simulink library "GOcontroll_Generic"  (R2023b)
settings: Solver=ode45  StartTime=0.0  StopTime=10.0  RelTol=1e-3  EnableMultiTasking=on
undefined symbols (not defined in the file or in its folder): C_CatOutPos, C_Cb1Pt10, Cb1Pt10_RAW_ERR_HIGH, Cb1Pt10_RAW_ERR_LOW, Cb1Pt10_SIG_ERR_HIGH, Cb1Pt10_SIG_ERR_LOW, Cb1Pt10_SIG_WAR_HIGH, Cb1Pt10_SIG_WAR_LOW, M_CatOutPos, Pres_0_20_bar_500_4500_mv_inv, SensorSignalSimulation, signal_x_RAW_ERR_HIGH, signal_x_RAW_ERR_LOW, signal_x_SIG_ERR_HIGH, signal_x_SIG_ERR_LOW, signal_x_SIG_WAR_HIGH, signal_x_SIG_WAR_LOW, signal_x_SPN, Valve1_ACTIVE_DUTY_CYCLE, Valve1_MAX_CURRENT, Valve1_MIN_CURRENT, Valve1_SPN
libraries: simulink x23, GOcontroll_Moduline_Target x20
(part 1 of 2)
settings Model: Creator=HANcoder  LastModifiedBy=maud
settings Model: ModifiedHistory=|
  | la_obwlf -- Thu Sep 01 12:12:55 2016 -- Version 0.33
  | 
  | 
  | 
  | 
  | 
  | 
  | la_obwlf -- Thu Sep 01 09:23:34 2016 -- Version 0.33
  | changed the version in the Base Sample Time block
  | 
  | 
  | 
  | la_obwlf -- Tue Aug 30 15:48:17 2016 -- Version 0.33
settings SolverCC: AlgebraicLoopSolver=TrustRegion
settings DataIOCC: LimitDataPoints=on  SaveFormat=Array  SignalLoggingSaveFormat=ModelDataLogs  ReturnWorkspaceOutputs=off
settings OptimizationCC: ExpressionDepthLimit=2147483647  LifeSpan=inf
settings DebuggingCC: UnderspecifiedInitializationDetection=Classic  MergeDetectMultiDrivingBlocksExec=none  SolverPrmCheckMsg=warning  FcnCallInpInsideContextMsg=warning  UnconnectedInputMsg=warning  UnconnectedOutputMsg=warning  UnconnectedLineMsg=warning  StateNameClashWarn=warning  SFUnexpectedBacktrackingDiag=warning  SFNoUnconditionalDefaultTransitionDiag=warning  SFExecutionAtInitializationDiag=none  ArithmeticOperatorsInVariantConditions=warning
settings HardwareCC: ProdBitPerPointer=32  ProdBitPerSizeT=32  ProdBitPerPtrDiffT=32  ProdLargestAtomicFloat=None  ProdIntDivRoundTo=Undefined  ProdEndianess=Unspecified  ProdWordSize=32  ProdHWDeviceType=32-bit Generic
settings ModelReferenceCC: EnableRefExpFcnMdlSchedulingChecks=on  PropagateSignalLabelsOutOfModel=off
settings SFSimCC: SimUseLocalCustomCode=off  CustomCodeUndefinedFunction=UseInterfaceOnly
settings RTWCC: RTWUseLocalCustomCode=off
settings CodeAppCC: StateflowObjectComments=on
settings GRTTargetCC: TargetLangStandard=C89/C90 (ANSI)  CombineOutputUpdateFcns=off  GRTInterface=on
settings ConfigComp: CovMetricSettings=dw  CovSaveCumulativeToWorkspaceVar=on  CovSaveSingleToWorkspaceVar=on  CovExternalEMLEnable=off  CovSFcnEnable=off

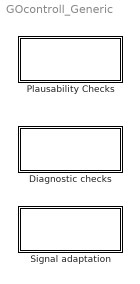
== system GOcontroll_Generic ==
  Diagnostic checks : Subsystem
      settings: MoveFcn=drawLogos
      mask Display: fprintf('Diagnostic');
  Plausability Checks : Subsystem
      settings: MoveFcn=drawLogos
      mask Display: fprintf('Plausability\n(deprecated)');
  Signal adaptation : Subsystem
      mask Display: fprintf('Signal adaptation');

== system GOcontroll_Generic/Diagnostic checks ==
  Actuator diagnostic : Subsystem  mask(Generic actuator diagnostic block){delay=1000, duration=2000, actuatorName=Valve1, spn=Valve1_SPN}
      mask prompts: delay "Start delay [ms]"; duration "Fault duration [ms]"; actuatorName "Actuator name:"
      mask help:
      | This block executes diagnostics on an actuator that goes into the block. The current during control is checked.
      |
      | It must be enabled via the enable input at the top to function, this can be a easy way to toggle diagnostics on or off.
      |
      | To use this block, error limits should be defined in the workspace. Several pre- and suffixes are needed to work with this block. For example:
      |
      | Base actuator name is: Valve1 (this will be the signal name in the mask)
      |
      | - Valve1_ACTIVE_DUTY_CYCLE (This is the dutycycle when the valve is controlles. in case a switch is used, use 1)
      | - Valve1_MIN_CURRENT (Current in mA that should be the minimal to control the valve)
      | - Valve1_MAX_CURRENT (Current in mA that should be the minimal to control the valve)
      |
      | Setting Diagnostic Trouble Code (DTC) in memory:
      |
      | Configure the SPN number corresponding to the signal in the workspace parameters as:
      | Valve1_SPN
      |
      | Output provide two uint8 signals in a bus holding the volatile and permanent fault flags.
      mask Callback actuatorName:
      | set_param(gcb, 'MaskSelfModifiable', 'on');
      | 
      | S = get_param(gcb,"actuatorName");
      | set_param(gcb + "/ActiveState",'const', S + "_ACTIVE_DUTY_CYCLE");
      | set_param(gcb + "/ActiveState2",'const', S + "_ACTIVE_DUTY_CYCLE");
      | set_param(gcb + "/MinimalCurrent",'const', S + "_MIN_CURRENT");
      | set_param(gcb + "/MaximalCurrent",'const', S + "_MAX_CURRENT");
      | 
      | set_param(gcb, 'spn', S + "_SPN");
      | 
      | % Set signal naming
      | P = get_param(gcb + "/Per",'PortHandles');
      | PerSubOut = P.Outport(1);
      | l1 = get_param(PerSubOut,'Line');
      | set_param(l1,'Name',"Per_" + S);
      | 
      | V = get_param(gcb + "/Vol",'PortHandles');
      | VolSubOut = V.Outport(1);
      | l1 = get_param(VolSubOut,'Line');
      | set_param(l1,'Name',"Vol_" + S);
      | 
      | try
      |     O = get_param(gcb,'PortHandles');
      |     PortOut = O.Outport(1);
      |     l1 = get_param(PortOut,'Line');
      |     set_param(l1,'Name',S);
      | end
      mask DialogControl ParameterGroupVar Prompt: Diagnostic parameters
      mask Display:
      | fprintf('%s\n SPN: %d',...
      |     actuatorName,spn);
      | 
      | port_label('input', 1, 'Reset');
      | port_label('input', 2, 'Duty cycle [0-1000]');
      | port_label('input', 3, 'Measured current [mA]');
      | 
      | text(2, 6, ert_linux_target_version());
  Diagnostic simulation : Subsystem  mask(Diagnostic simulation){signalName=Cb1Pt10, sensorCurveText=Pres_0_20_bar_500_4500_mv_inv, sensorCurve=Pres_0_20_bar_500_4500_mv_inv}
      mask prompts: signalName "Signal"; sensorCurveText "Sensor curve"
      mask help:
      | This block works together with the "Signal adaptation" and "Signal diagnostic" blocks to provide an easy way to test the setting of diagnostic codes for analogue inputs.
      |
      | It needs both of those blocks to be properly set up in the model along with their workspace variables. Then the Simulation variable of this signal must be set to 1.
      |
      | A diagnostic scenario can then be injected:
      | == 1/default: normal operation
      | == 2: low voltage
      | == 3: high voltage
      | == 4: too low error
      | == 5: too high error
      | == 6: too low warning
      | == 7: too high warning
      |
      | To simulate this it requires an extra lookup table which is the inverse of the normal signal lookup table, it should transfor the real world value back into the raw input.
      mask Callback signalName:
      | set_param(gcb, 'MaskSelfModifiable', 'on');
      | 
      | S = get_param(gcb,"signalName");
      |  set_param(gcb + "/LowVoltage", 'Value', S + "_RAW_ERR_LOW -1");
      |  set_param(gcb + "/HighVoltage", 'Value', S + "_RAW_ERR_HIGH +1");
      |  set_param(gcb + "/LowWarning",  'Value',S + "_SIG_WAR_LOW -1");
      |  set_param(gcb + "/HighWarning", 'Value', S + "_SIG_WAR_HIGH +1");
      |  set_param(gcb + "/LowError", 'Value', S + "_SIG_ERR_LOW -1");
      |  set_param(gcb + "/HighError", 'Value', S + "_SIG_ERR_HIGH +1");
      |  set_param(gcb + "/Normal", 'Value', "C_" + S);
      | 
      | % Set Goto tags depending on signal naming
      | set_param(gcb + "/ToRaw","GotoTag","RawSim_" + S);
      | set_param(gcb, "sensorCurve", get_param(gcb,"sensorCurveText"));
      mask Display:
      | fprintf('%s', signalName);
      | 
      | text(2, 6, ert_linux_target_version());
  Generic diagnostic : Subsystem  mask(Generic actuator diagnostic block){delay=1000, duration=2000, naming=Valve2, spn=1234, fmi=(0) Data valid but above normal operational range, most severe level (3)}
      mask prompts: delay "Start delay [ms]"; duration "Fault duration [ms]"; spn "SPN number"; fmi "Failure Mode Indicator"
      mask help:
      | A simple diagnostic helper, diagnostics start after "Start delay" and then if trigger == 1 for "Fault duration" it will write the fault code to memory.
      |
      | Once the trigger drops to 0 again, the volatile output will also go back to 0, but the persistant output will remain at 1. Untill the reset input is applied, this will also reset the persistant output. Note that this will not delete the code from memory.
      |
      | The naming parameter is non functional but helps by naming the output signals and being displayed in the mask.
      mask Callback naming:
      | set_param(gcb, 'MaskSelfModifiable', 'on');
      | 
      | S = get_param(gcb,"naming");
      | 
      | % Set signal naming
      | try
      |     P = get_param(gcb,'PortHandles');
      |     OutputPort1 = P.Outport(1);
      |     l1 = get_param(OutputPort1,'Line');
      |     set_param(l1,'Name',"Per_" + S);
      | 
      |     OutputPort2 = P.Outport(2);
      |     l1 = get_param(OutputPort2,'Line');
      |     set_param(l1,'Name',"Vol_" + S);
      | end
      mask TypeOptions spn: Store diagnostic code/spn
      mask TypeOptions fmi: Store diagnostic code/fmi
      mask DialogControl ParameterGroupVar Prompt: Diagnostic parameters
      mask Display:
      | fprintf('%s\n\nDTC serverity: %d\nSPN: %d',...
      |     naming,fmi,spn);
      | 
      | port_label('input', 1, 'Reset');
      | port_label('input', 2, 'Trigger');
      | 
      | port_label('output', 1, 'Persistant flag');
      | port_label('output', 2, 'Volatile flag');
      | 
      | text(2, 6, ert_linux_target_version());
  Signal diagnostic : Subsystem  mask(Generic Signal diagnostic block){delay=1000, duration=1000, signalName=signal_x, spn=signal_x_SPN}
      mask prompts: delay "Start delay [ms]"; duration "Fault duration [ms]"; signalName "Signal name:"
      mask help:
      | This block executes diagnostics on a signal that goes into the block. Both sensor voltage and signal thersholds are checked.
      |
      | It must be enabled via the enable input at the top to function, this can be a easy way to toggle diagnostics on or off.
      |
      | To use this block, error and warning limits should be defined in the workspace. Several pre- and suffixes are needed to work with this block. For example:
      |
      | Base signal name is: Coolant_Pt1 (this will be the signal name in the mask)
      |
      | - Coolant_Pt1_RAW_ERR_LOW (low voltage error)
      | - Coolant_Pt1_RAW_ERR_HIGH (high voltage error)
      | - Coolant_Pt1_SIG_WAR_LOW (Low warning signal threshold)
      | - Coolant_Pt1_SIG_WAR_HIGH (High warning signal threshold)
      | - Coolant_Pt1_SIG_ERR_LOW (Low error signal threshold)
      | - Coolant_Pt1 _SIG_ERR_HIGH (High error signal threshold)
      |
      | Setting Diagnostic Trouble Code (DTC) in memory:
      |
      | Configure the SPN number corresponding to the signal in the workspace parameters as:
      | Coolant_Pt1_SPN
      |
      | Output provide two uint8 signals in a bus holding the volatile and permanent fault flags.
      mask Callback signalName:
      | set_param(gcb, 'MaskSelfModifiable', 'on');
      | 
      | S = get_param(gcb,"signalName");
      | set_param(gcb + "/LowVoltage",'const', S + "_RAW_ERR_LOW");
      | set_param(gcb + "/HighVoltage",'const', S + "_RAW_ERR_HIGH");
      | set_param(gcb + "/LowWarning",'const', S + "_SIG_WAR_LOW");
      | set_param(gcb + "/HighWarning",'const', S + "_SIG_WAR_HIGH");
      | set_param(gcb + "/LowError",'const', S + "_SIG_ERR_LOW");
      | set_param(gcb + "/HighError",'const', S + "_SIG_ERR_HIGH");
      | 
      | set_param(gcb,'spn', S + "_SPN");
      | 
      | % Set signal naming
      | P = get_param(gcb + "/Per",'PortHandles');
      | PerSubOut = P.Outport(1);
      | l1 = get_param(PerSubOut,'Line');
      | set_param(l1,'Name',"Per_" + S);
      | 
      | V = get_param(gcb + "/Vol",'PortHandles');
      | VolSubOut = V.Outport(1);
      | l1 = get_param(VolSubOut,'Line');
      | set_param(l1,'Name',"Vol_" + S);
      | 
      | try
      |     O = get_param(gcb,'PortHandles');
      |     PortOut = O.Outport(1);
      |     l1 = get_param(PortOut,'Line');
      |     set_param(l1,'Name',S);
      | end
      mask DialogControl ParameterGroupVar Prompt: Diagnostic parameters
      mask Display:
      | fprintf('%s\nSPN: %d',...
      |     signalName,spn);
      | 
      | port_label('input', 1, 'Reset');
      | port_label('input', 2, 'RAW signal');
      | port_label('input', 3, 'Physical signal');
      | 
      | text(2, 6, ert_linux_target_version());

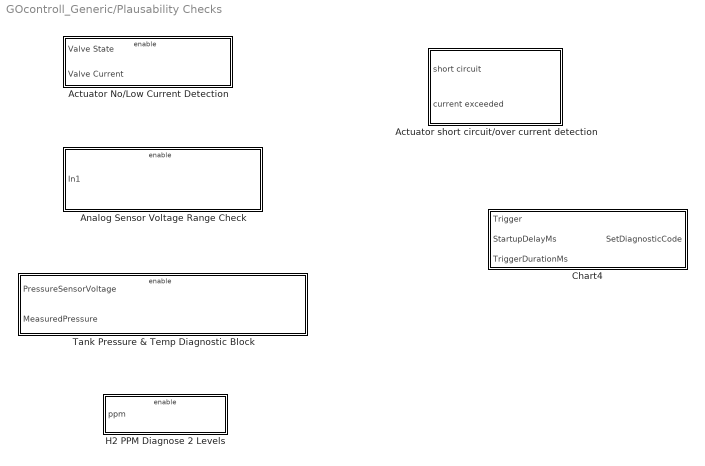
== system GOcontroll_Generic/Plausability Checks ==
  Actuator No/Low Current Detection : Subsystem  TreatAsAtomicUnit=on  mask{Signal=1}
      mask prompts: Signal "Actuator Number"
      mask Display: fprintf("Actuator no/low current detection\nActuator number: %d",Signal);
  Actuator short circuit/over current detection : Subsystem  mask{Signal=1, BaseNum=0}
      mask prompts: Signal "Actuator Number"; BaseNum "Fault Code Base Number"
      mask Display:
      | fprintf("Actuator short circuit/over current detection\nActuator number: %d",Signal);
      | port_label("input", 1, "Short circuit");
      | port_label("input", 2, "Current exceeded");
  Analog Sensor Voltage Range Check : Subsystem  mask{Signal=1, FaultCodeBase=0, TC=0, DSDelay=0, MinFaultDur=0, MinVoltage=0, MaxVoltage=0}
      mask prompts: Signal "Sensor Number"; FaultCodeBase "Fault Code Base Number"; TC "Trouble Code"; DSDelay "Diagnostics Startup Delay"; MinFaultDur "Minimum Fault Duration"; MinVoltage "Minimum Sensor Voltage"; MaxVoltage "Maximum Sensor Voltage"
      mask Display: fprintf('Analog Sensor Voltage Diagnostics\nSignal Code: %d',Signal);
  Chart4 : Stateflow chart  TreatAsAtomicUnit=on
  H2 PPM Diagnose 2 Levels : Subsystem  TreatAsAtomicUnit=on  mask{Signal=1, DSDelay=0, MinFaultDur=0, FaultBaseCode=0, TC=0}
      mask prompts: Signal "Sensor Number"; DSDelay "Diagnostic Startup Delay"; MinFaultDur "Minimal Fault Duration"; FaultBaseCode "Fault Code Base Number"; TC "Trouble Code"
      mask Display: fprintf('H2 PPM Check\nSensor Number: %d',Signal);
  Tank Pressure & Temp Diagnostic Block : Subsystem  mask{Signal=1, Cent=0, MinFaultDuration=0, DSDelay=0, MinVoltage=0, MaxVoltage=0, HighLimit1=0, HighLimit2=0, LowLimit1=0, LowLimit2=0}
      mask prompts: Cent "Fault Code Centenial value"; MinFaultDuration "Minimal Fault Duration"; DSDelay "Diagnostic Startup Delay"; MinVoltage "Minimum Sensor Voltage"; MaxVoltage "Maximum Sensor Voltage"; HighLimit1 "High Limit Level 1"; HighLimit2 "High Limit Level 2"; LowLimit1 "Low Limit Level 1"; LowLimit2 "Low Limit Level 2"
      mask help:
      | Single sensor diagnosis block for temperature and pressure sensors that come in the form:
      | 2 levels of too high and too low pressur or temp etc
      | sensor over and under voltage detection.
      mask Help:
      | Signal = number of unit it is on: Tank 1 or GHU 2 etc.
      | Fault Code Centenial Value = if a fault code is 170x11, x is the centenial value.
      | 
      | Minimal Fault duration = the time a fault needs to persist for it to trigger a diagnostic code
      | Diagnostic Startup Delay = a delay before the diagnostic system starts doing diagnostics.
      | 
      | Minimum Sensor Voltage = the lowest the voltage of a sensor is allowed to be before triggering a fault
      | Maximum Sensor Voltage = the highest the voltage of a sensor is allowed to be before triggering a fault
      | 
      | these voltage measurements are done in miliVolts
      | 
      | High Limit Level 1 = The value read by the sensor triggering the first x value is too high warning.
      | High Limit Level 2 = the value read by the sensor triggering the the warning with required action.
      | 
      | Low Limit Level 1 = The value read by the sensor triggering the first x value is too low warning.
      | Low Limit Level 2 = the value read by the sensor triggering the the warning with required action.
      | 
      | these measurements are done by the system in their unit values, celsius for temp, bar for pressure.
      mask Display: fprintf('Pressure and Temperature Sensor Diagnostics\nSignal Code: %d',Signal);

== system GOcontroll_Generic/Signal adaptation ==
  Signal adaptation : Subsystem  mask(Signal adaptation){signalName=CatOutPos, simulationSource=SensorSignalSimulation}
      mask prompts: signalName "Signal name:"; simulationSource "Simulation source"
      mask help:
      | This block helps with setting up a sensor, it integrates a lookup table, sensor overrides for XCP and the possibility to simulate the signal.
      |
      | It depends on a couple of workspace parameters, for example if your signal is to called "temperature1" it will expect three workspace parameters: "C_temperature1", "M_temperature1", "temperature1_Table".
      |
      | This first one is the override value as a physical real world unit equal to the output of the lookup table, The "M_signal name" variable determines whether the override is active or not, 0 == use incoming signal, > 0 == use override value from "C_signal name". These should be "exported global" so they can be manipulatied via XCP.
      |
      | The last one is the sensor lookup table.
      |
      | The Simulation source variable can have three effects:
      | == 1: Simulate the Raw input value and run it through the lookup table.
      | == 2: Simulate the physical value which will go to the output directly. Note that this will not give a valid output on the RAW signal output.
      | == !1 and !2: Don't simulate, use block input signal.
      mask init:
      | set_param(gcb, 'MaskSelfModifiable', 'on');
      | 
      | % Set manual Overrides
      | S = get_param(gcb,"signalName");
      | set_param(gcb + "/Manual", 'Value', "M_" + S)
      | set_param(gcb + "/Control", 'Value', "C_" + S)
      | 
      | % Define raw to physics curve
      | set_param(gcb + "/RawToPhysic", 'LookupTableObject', S + "_Table")
      | 
      | try
      |     % Set signal naming 
      |     P = get_param(gcb,'PortHandles');
      |     outport1 = P.Outport(1);
      |     outport2 = P.Outport(2);
      |     l1 = get_param(outport1,'Line');
      |     l2 = get_param(outport2,'Line');
      |     set_param(l1,'Name',S);
      |     set_param(l2,'Name',S);
      | end
      | 
      | % Set Goto tags depending on signal naming
      | set_param(gcb + "/FromRaw","GotoTag","RawSim_" + S);
      | set_param(gcb + "/FromPhys","GotoTag","PhysSim_" + S);
      | 
      | % Set signal specific name of block
      | G = get_param(gcb,"simulationSource");
      | set_param(gcb + "/Simulation1","Value",G);
      | set_param(gcb + "/Simulation2","Value",G);
      mask Callback signalName:
      | set_param(gcb, 'MaskSelfModifiable', 'on');
      | 
      | % Set manual Overrides
      | S = get_param(gcb,"signalName");
      | set_param(gcb + "/Manual", 'Value', "M_" + S)
      | set_param(gcb + "/Control", 'Value', "C_" + S)
      | 
      | % Define raw to physics curve
      | set_param(gcb + "/RawToPhysic", 'LookupTableObject', S + "_Table")
      | 
      | try
      |     % Set signal naming
      |     P = get_param(gcb,'PortHandles');
      |     outport1 = P.Outport(1);
      |     outport2 = P.Outport(2);
      |     l1 = get_param(outport1,'Line');
      |     l2 = get_param(outport2,'Line');
      |     set_param(l1,'Name',S);
      |     set_param(l2,'Name',S);
      | end
      | 
      | % Set Goto tags depending on signal naming
      | set_param(gcb + "/FromRaw","GotoTag","RawSim_" + S);
      | set_param(gcb + "/FromPhys","GotoTag","PhysSim_" + S);
      | 
      | % Set signal specific name of block
      | G = get_param(gcb,"simulationSource");
      | set_param(gcb + "/Simulation1","Value",G);
      | set_param(gcb + "/Simulation2","Value",G);
      mask Display:
      | fprintf('%s\nCurve: %s\n\nGlobal Goto:    %s  -  %s',signalName,...
      |     signalName + "_Table","RawSim_" + signalName,"RawPhys_" + signalName);
      | port_label('output', 1, 'Physical');
      | port_label('output', 2, 'RAW');
      | port_label('input', 1, 'RAW input');
      | 
      | text(2, 6, ert_linux_target_version());
  Signal adaptation digital : Subsystem  mask(Signal adaptation digital){signalName=CatOutPos, simulationSource=SensorSignalSimulation, OffSwitchValue=1500, OnSwitchValue=3500}
      mask prompts: signalName "Signal name:"; simulationSource "Simulation source"; OffSwitchValue "Simulink:blkprm_prompts:RelaySwitchOffPoint"; OnSwitchValue "Simulink:blkprm_prompts:RelaySwitchOnPoint"
      mask help:
      | This block helps with setting up a sensor, it integrates a relay for hysteresis, sensor overrides for XCP and the possibility to simulate the signal.
      |
      | It depends on a couple of workspace parameters, for example if your signal is to called "deviceOn" it will expect two workspace parameters: "C_deviceOn", "M_deviceOn".
      |
      | This first one is the override value, while this is boolean, the uint8 datatype is used, The "M_signal name" variable determines whether the override is active or not, 0 == use incoming signal, > 0 == use override value from "C_signal name". These should be "exported global" so they can be manipulatied via XCP
      mask init:
      | set_param(gcb, 'MaskSelfModifiable', 'on');
      | 
      | % Set manual Overrides
      | S = get_param(gcb,"signalName");
      | set_param(gcb + "/Manual", 'Value', "M_" + S)
      | set_param(gcb + "/Control", 'Value', "C_" + S)
      | 
      | try
      |     % Set signal naming 
      |     P = get_param(gcb,'PortHandles');
      |     outport1 = P.Outport(1);
      |     outport2 = P.Outport(2);
      |     l1 = get_param(outport1,'Line');
      |     l2 = get_param(outport2,'Line');
      |     set_param(l1,'Name',S);
      |     set_param(l2,'Name',S);
      | end
      | 
      | % Set Goto tags depending on signal naming
      | set_param(gcb + "/FromRaw","GotoTag","RawSim_" + S);
      | set_param(gcb + "/FromPhys","GotoTag","PhysSim_" + S);
      | 
      | % Set signal specific name of block
      | G = get_param(gcb,"simulationSource");
      | set_param(gcb + "/Simulation1","Value",G);
      | set_param(gcb + "/Simulation2","Value",G);
      mask Callback signalName:
      | set_param(gcb, 'MaskSelfModifiable', 'on');
      | 
      | % Set manual Overrides
      | S = get_param(gcb,"signalName");
      | set_param(gcb + "/Manual", 'Value', "M_" + S)
      | set_param(gcb + "/Control", 'Value', "C_" + S)
      | 
      | try
      |     % Set signal naming
      |     P = get_param(gcb,'PortHandles');
      |     outport1 = P.Outport(1);
      |     outport2 = P.Outport(2);
      |     l1 = get_param(outport1,'Line');
      |     l2 = get_param(outport2,'Line');
      |     set_param(l1,'Name',S);
      |     set_param(l2,'Name',S);
      | end
      | 
      | % Set Goto tags depending on signal naming
      | set_param(gcb + "/FromRaw","GotoTag","RawSim_" + S);
      | set_param(gcb + "/FromPhys","GotoTag","PhysSim_" + S);
      | 
      | % Set signal specific name of block
      | G = get_param(gcb,"simulationSource");
      | set_param(gcb + "/Simulation1","Value",G);
      | set_param(gcb + "/Simulation2","Value",G);
      mask TypeOptions OffSwitchValue: Relay/OffSwitchValue
      mask TypeOptions OnSwitchValue: Relay/OnSwitchValue
      mask DialogControl OffSwitchValue Prompt: Switch off point:
      mask DialogControl OnSwitchValue Prompt: Switch on point:
      mask Display:
      | fprintf('%s\nCurve: %s\n\nGlobal Goto:    %s',signalName,...
      |     "RawSim_" + signalName,"RawPhys_" + signalName);
      | port_label('output', 1, 'Physical');
      | port_label('output', 2, 'RAW');
      | port_label('input', 1, 'RAW input');
      | 
      | text(2, 6, ert_linux_target_version());

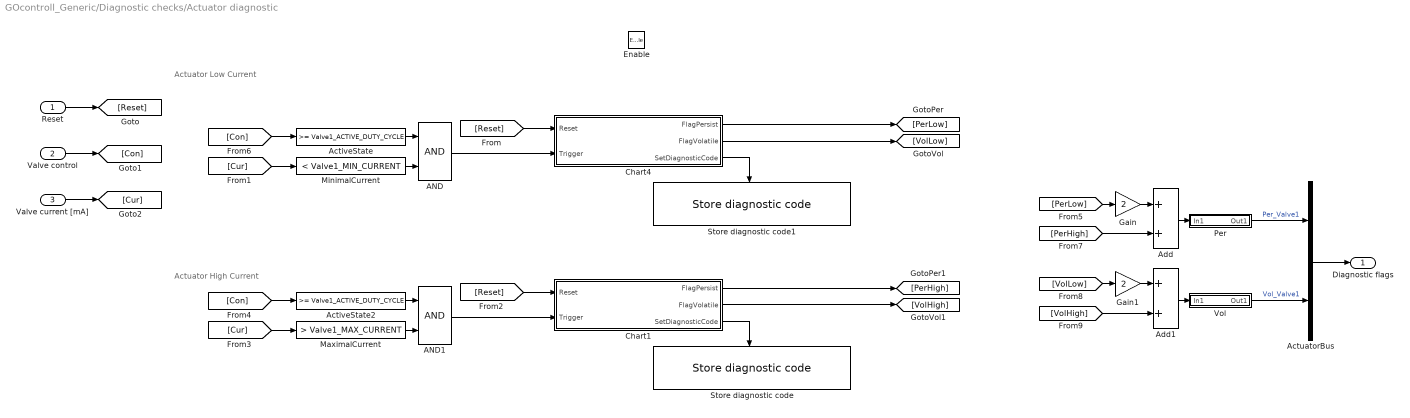
== system GOcontroll_Generic/Diagnostic checks/Actuator diagnostic ==
  note: Actuator High Current
  note: Actuator Low Current
  Reset : Inport
  "Valve control " : Inport  Port=2
  Valve current [mA] : Inport  Port=3
  Enable : EnablePort
  AND : Logic  AllPortsSameDT=off  OutDataTypeStr=boolean
  AND1 : Logic  AllPortsSameDT=off  OutDataTypeStr=boolean
  ActiveState : simulink/Logic and Bit Operations/Compare To Constant  relop=>=  const=Valve1_ACTIVE_DUTY_CYCLE  OutDataTypeStr=boolean
  ActiveState2 : simulink/Logic and Bit Operations/Compare To Constant  relop=>=  const=Valve1_ACTIVE_DUTY_CYCLE  OutDataTypeStr=boolean
  ActuatorBus : BusCreator  Inputs=2
  Add : Sum  OutDataTypeStr=uint8
  Add1 : Sum  AccumDataTypeStr=uint8
  Chart1 : Stateflow chart  TreatAsAtomicUnit=on
  Chart4 : Stateflow chart  TreatAsAtomicUnit=on
  Gain : Gain  Gain=2  OutDataTypeStr=uint8
  Gain1 : Gain  Gain=2  OutDataTypeStr=uint8
  MaximalCurrent : simulink/Logic and Bit Operations/Compare To Constant  relop=>  const=Valve1_MAX_CURRENT  OutDataTypeStr=boolean
  MinimalCurrent : simulink/Logic and Bit Operations/Compare To Constant  relop=<  const=Valve1_MIN_CURRENT  OutDataTypeStr=boolean
  Per : Subsystem
  Store diagnostic code : GOcontroll_Moduline_Target/Memory store/Diagnostic to memory/Store diagnostic code  spn=spn  fmi=(6) Current above normal, or grounded circuit  TriggerType=rising
      settings: SourceProductName=GOcontroll Moduline
  Store diagnostic code1 : GOcontroll_Moduline_Target/Memory store/Diagnostic to memory/Store diagnostic code  spn=spn  fmi=(5) Current below normal, or open circuit  TriggerType=rising
      settings: SourceProductName=GOcontroll Moduline
  Vol : Subsystem
  Diagnostic flags : Outport  OutputWhenDisabled=reset  InitialOutput=[0]
  wires:
  [PerHigh] -> Add/2
  [VolHigh] -> Add1/2
  Gain1/1 -> Add1/1
  [VolLow] -> Gain1/1
  Gain/1 -> Add/1
  [PerLow] -> Gain/1
  Chart4/2(FlagVolatile) -> [VolLow]
  Chart4/1(FlagPersist) -> [PerLow]
  Add1/1 -> Vol/1(In1)
  Vol/1(Out1) -> ActuatorBus/2  "Vol_Valve1"
  Per/1(Out1) -> ActuatorBus/1  "Per_Valve1"
  Add/1 -> Per/1(In1)
  [Cur] -> MaximalCurrent/1
  ActiveState2/1 -> AND1/1
  Chart1/3(SetDiagnosticCode) -> Store diagnostic code/Trigger
  AND1/1 -> Chart1/2(Trigger)
  [Reset] -> Chart1/1(Reset)
  Chart1/1(FlagPersist) -> [PerHigh]
  [Con] -> ActiveState2/1
  Chart1/2(FlagVolatile) -> [VolHigh]
  MaximalCurrent/1 -> AND1/2
  ActuatorBus/1 -> Diagnostic flags/1
  Valve current [mA]/1 -> [Cur]
  "Valve control "/1 -> [Con]
  [Reset] -> Chart4/1(Reset)
  Reset/1 -> [Reset]
  AND/1 -> Chart4/2(Trigger)
  Chart4/3(SetDiagnosticCode) -> Store diagnostic code1/Trigger
  [Con] -> ActiveState/1
  [Cur] -> MinimalCurrent/1
  MinimalCurrent/1 -> AND/2
  ActiveState/1 -> AND/1

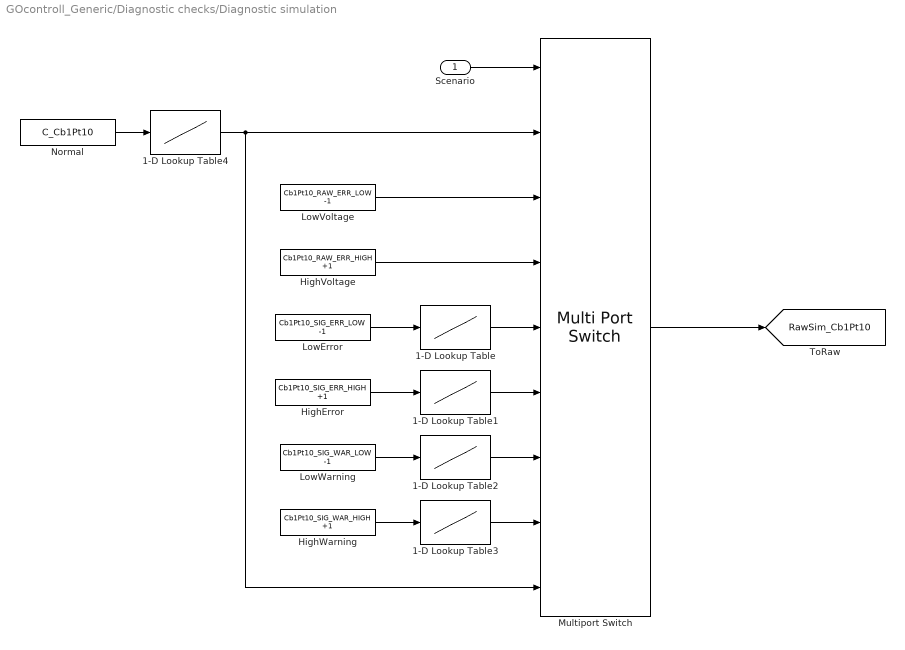
== system GOcontroll_Generic/Diagnostic checks/Diagnostic simulation ==
  Scenario : Inport
  1-D Lookup Table{,1..4} (5 alike) : Lookup_n-D  NumberOfTableDimensions=1  DataSpecification=Lookup table object  LookupTableObject=sensorCurve  BreakpointsForDimension1=[-5:5]  Table=tanh([-5:5])  ExtrapMethod=Clip  InternalRulePriority=Speed  RndMeth=Simplest
  HighError : Constant  Value=Cb1Pt10_SIG_ERR_HIGH +1
  HighVoltage : Constant  Value=Cb1Pt10_RAW_ERR_HIGH +1  OutDataTypeStr=uint16
  HighWarning : Constant  Value=Cb1Pt10_SIG_WAR_HIGH +1
  LowError : Constant  Value=Cb1Pt10_SIG_ERR_LOW -1
  LowVoltage : Constant  Value=Cb1Pt10_RAW_ERR_LOW -1  VectorParams1D=off  OutDataTypeStr=int16
  LowWarning : Constant  Value=Cb1Pt10_SIG_WAR_LOW -1  OutDataTypeStr=single
  Multiport Switch : MultiPortSwitch  Inputs=7  DataPortForDefault=Additional data port  SaturateOnIntegerOverflow=off  InputSameDT=off
  Normal : Constant  Value=C_Cb1Pt10  VectorParams1D=off
  tag scope: RawSim_Cb1Pt10=global
  wires:
  HighError/1 -> 1-D Lookup Table1/1
  LowError/1 -> 1-D Lookup Table/1
  HighWarning/1 -> 1-D Lookup Table3/1
  LowWarning/1 -> 1-D Lookup Table2/1
  1-D Lookup Table/1 -> Multiport Switch/5
  1-D Lookup Table3/1 -> Multiport Switch/8
  1-D Lookup Table2/1 -> Multiport Switch/7
  HighVoltage/1 -> Multiport Switch/4
  Scenario/1 -> Multiport Switch/1
  Multiport Switch/1 -> [RawSim_Cb1Pt10]
  LowVoltage/1 -> Multiport Switch/3
  1-D Lookup Table1/1 -> Multiport Switch/6
  1-D Lookup Table4/1 -> Multiport Switch/9, Multiport Switch/2
  Normal/1 -> 1-D Lookup Table4/1

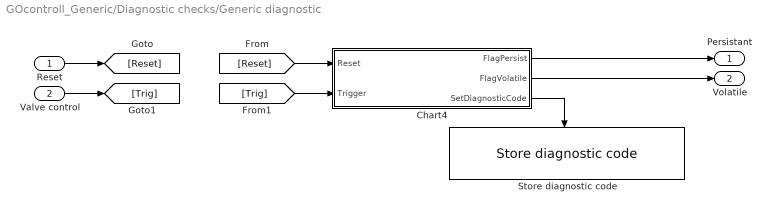
== system GOcontroll_Generic/Diagnostic checks/Generic diagnostic ==
  Reset : Inport
  "Valve control " : Inport  Port=2
  Chart4 : Stateflow chart  TreatAsAtomicUnit=on
  Store diagnostic code : GOcontroll_Moduline_Target/Memory store/Diagnostic to memory/Store diagnostic code  spn=spn  fmi=(0) Data valid but above normal operational range, most severe level (3)  TriggerType=rising
      settings: SourceProductName=GOcontroll Moduline
  Persistant : Outport
  Volatile : Outport  Port=2
  wires:
  Chart4/2(FlagVolatile) -> Volatile/1
  Chart4/1(FlagPersist) -> Persistant/1
  "Valve control "/1 -> [Trig]
  [Reset] -> Chart4/1(Reset)
  Reset/1 -> [Reset]
  [Trig] -> Chart4/2(Trigger)
  Chart4/3(SetDiagnosticCode) -> Store diagnostic code/Trigger

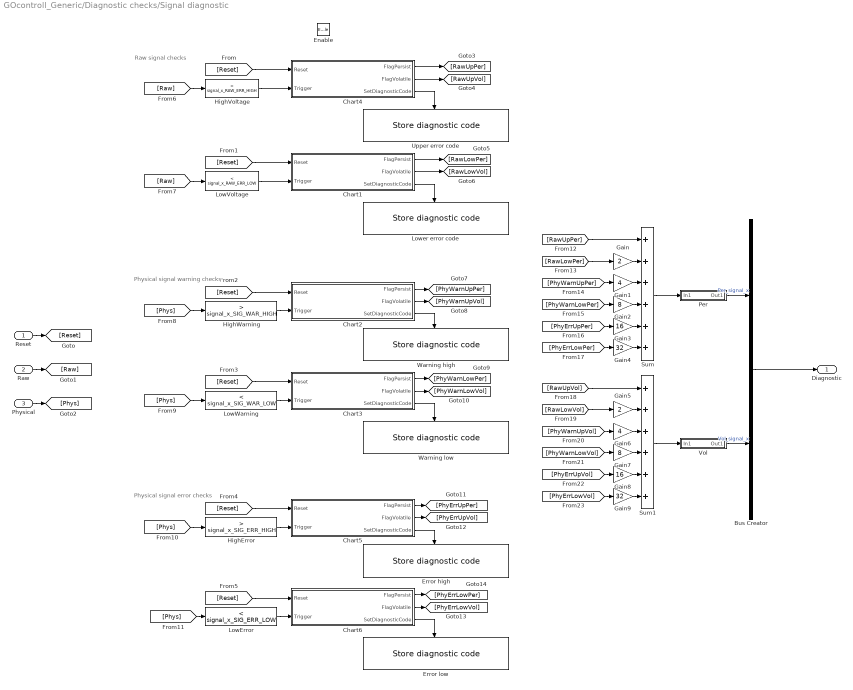
== system GOcontroll_Generic/Diagnostic checks/Signal diagnostic ==
  note: Physical signal error checks
  note: Raw signal checks
  note: Physical signal warning checks
  Reset : Inport
  Raw : Inport  Port=2
  Physical : Inport  Port=3
  Enable : EnablePort
  Bus Creator : BusCreator  Inputs=2
  Chart1 : Stateflow chart  TreatAsAtomicUnit=on
  Chart2 : Stateflow chart  TreatAsAtomicUnit=on
  Chart3 : Stateflow chart  TreatAsAtomicUnit=on
  Chart4 : Stateflow chart  TreatAsAtomicUnit=on
  Chart5 : Stateflow chart  TreatAsAtomicUnit=on
  Chart6 : Stateflow chart  TreatAsAtomicUnit=on
  Error high : GOcontroll_Moduline_Target/Memory store/Diagnostic to memory/Store diagnostic code  Tag=HANcoder_GOcontroll_Moduline_IV  spn=spn  fmi=(0) Data valid but above normal operational range, most severe level (3)  TriggerType=rising
      settings: SourceProductName=GOcontroll Moduline
  Error low : GOcontroll_Moduline_Target/Memory store/Diagnostic to memory/Store diagnostic code  Tag=HANcoder_GOcontroll_Moduline_IV  spn=spn  fmi=(1) Data valid but below normal operational range, most severe level (3)  TriggerType=rising
      settings: SourceProductName=GOcontroll Moduline
  Gain : Gain  Gain=2
  Gain1 : Gain  Gain=4
  Gain2 : Gain  Gain=8
  Gain3 : Gain  Gain=16
  Gain4 : Gain  Gain=32
  Gain5 : Gain  Gain=2
  Gain6 : Gain  Gain=4
  Gain7 : Gain  Gain=8
  Gain8 : Gain  Gain=16
  Gain9 : Gain  Gain=32
  HighError : simulink/Logic and Bit Operations/Compare To Constant  relop=>  const=signal_x_SIG_ERR_HIGH  OutDataTypeStr=boolean
  HighVoltage : simulink/Logic and Bit Operations/Compare To Constant  relop=>  const=signal_x_RAW_ERR_HIGH  OutDataTypeStr=boolean
  HighWarning : simulink/Logic and Bit Operations/Compare To Constant  relop=>  const=signal_x_SIG_WAR_HIGH  OutDataTypeStr=boolean
  LowError : simulink/Logic and Bit Operations/Compare To Constant  relop=<  const=signal_x_SIG_ERR_LOW  OutDataTypeStr=boolean
  LowVoltage : simulink/Logic and Bit Operations/Compare To Constant  relop=<  const=signal_x_RAW_ERR_LOW  OutDataTypeStr=boolean
  LowWarning : simulink/Logic and Bit Operations/Compare To Constant  relop=<  const=signal_x_SIG_WAR_LOW  OutDataTypeStr=boolean
  Lower error code : GOcontroll_Moduline_Target/Memory store/Diagnostic to memory/Store diagnostic code  Tag=HANcoder_GOcontroll_Moduline_IV  spn=spn  fmi=(4) Voltage below normal, or shorted to low source  TriggerType=rising
      settings: SourceProductName=GOcontroll Moduline
  Per : Subsystem
  Sum : Sum  Inputs=++++++  OutDataTypeStr=uint8
  Sum1 : Sum  Inputs=++++++  OutDataTypeStr=uint8
  Upper error code : GOcontroll_Moduline_Target/Memory store/Diagnostic to memory/Store diagnostic code  Tag=HANcoder_GOcontroll_Moduline_IV  spn=spn  fmi=(3) Voltage above normal, or shorted to high source  TriggerType=rising
      settings: SourceProductName=GOcontroll Moduline
  Vol : Subsystem
  Warning high : GOcontroll_Moduline_Target/Memory store/Diagnostic to memory/Store diagnostic code  Tag=HANcoder_GOcontroll_Moduline_IV  spn=spn  fmi=(15) Data valid but above normal range: least severe level (1)  TriggerType=rising
      settings: SourceProductName=GOcontroll Moduline
  Warning low : GOcontroll_Moduline_Target/Memory store/Diagnostic to memory/Store diagnostic code  Tag=HANcoder_GOcontroll_Moduline_IV  spn=spn  fmi=(17) Data valid but below normal range: least severe level (1)  TriggerType=rising
      settings: SourceProductName=GOcontroll Moduline
  Diagnostic : Outport  OutputWhenDisabled=reset  InitialOutput=[0]
  wires:
  Per/1(Out1) -> Bus Creator/1  "Per_signal_x"
  Vol/1(Out1) -> Bus Creator/2  "Vol_signal_x"
  Bus Creator/1 -> Diagnostic/1
  [PhyErrLowVol] -> Gain9/1
  [PhyErrUpVol] -> Gain8/1
  [PhyWarnUpVol] -> Gain6/1
  [PhyWarnLowVol] -> Gain7/1
  [RawLowVol] -> Gain5/1
  Gain8/1 -> Sum1/5
  Gain7/1 -> Sum1/4
  Gain5/1 -> Sum1/2
  Gain6/1 -> Sum1/3
  Sum1/1 -> Vol/1(In1)
  Gain9/1 -> Sum1/6
  [RawUpVol] -> Sum1/1
  Sum/1 -> Per/1(In1)
  [PhyErrLowPer] -> Gain4/1
  [PhyErrUpPer] -> Gain3/1
  [PhyWarnLowPer] -> Gain2/1
  [PhyWarnUpPer] -> Gain1/1
  Gain2/1 -> Sum/4
  Gain3/1 -> Sum/5
  Gain4/1 -> Sum/6
  Gain1/1 -> Sum/3
  Gain/1 -> Sum/2
  [RawLowPer] -> Gain/1
  [RawUpPer] -> Sum/1
  Chart6/2(FlagVolatile) -> [PhyErrLowVol]
  Chart6/1(FlagPersist) -> [PhyErrLowPer]
  Chart5/2(FlagVolatile) -> [PhyErrUpVol]
  Chart5/1(FlagPersist) -> [PhyErrUpPer]
  Chart3/2(FlagVolatile) -> [PhyWarnLowVol]
  Chart3/1(FlagPersist) -> [PhyWarnLowPer]
  Chart2/2(FlagVolatile) -> [PhyWarnUpVol]
  Chart2/1(FlagPersist) -> [PhyWarnUpPer]
  Chart1/2(FlagVolatile) -> [RawLowVol]
  Chart1/1(FlagPersist) -> [RawLowPer]
  Chart4/2(FlagVolatile) -> [RawUpVol]
  Chart4/1(FlagPersist) -> [RawUpPer]
  [Phys] -> LowError/1
  [Phys] -> HighError/1
  [Phys] -> LowWarning/1
  [Phys] -> HighWarning/1
  Physical/1 -> [Phys]
  [Raw] -> LowVoltage/1
  [Raw] -> HighVoltage/1
  Raw/1 -> [Raw]
  [Reset] -> Chart6/1(Reset)
  [Reset] -> Chart5/1(Reset)
  [Reset] -> Chart3/1(Reset)
  [Reset] -> Chart2/1(Reset)
  [Reset] -> Chart1/1(Reset)
  [Reset] -> Chart4/1(Reset)
  Reset/1 -> [Reset]
  LowError/1 -> Chart6/2(Trigger)
  HighError/1 -> Chart5/2(Trigger)
  Chart5/3(SetDiagnosticCode) -> Error high/Trigger
  Chart6/3(SetDiagnosticCode) -> Error low/Trigger
  Chart3/3(SetDiagnosticCode) -> Warning low/Trigger
  LowWarning/1 -> Chart3/2(Trigger)
  Chart2/3(SetDiagnosticCode) -> Warning high/Trigger
  HighWarning/1 -> Chart2/2(Trigger)
  Chart1/3(SetDiagnosticCode) -> Lower error code/Trigger
  LowVoltage/1 -> Chart1/2(Trigger)
  HighVoltage/1 -> Chart4/2(Trigger)
  Chart4/3(SetDiagnosticCode) -> Upper error code/Trigger

== system GOcontroll_Generic/Plausability Checks/Actuator No//Low Current Detection ==
  Valve State : Inport
  Valve Current : Inport  Port=2
  Enable : EnablePort
  Chart : Stateflow chart  TreatAsAtomicUnit=on
  Terminator : Terminator
  wires:
  Chart/1(SetDiagnosticCode) -> Terminator/1
  Valve State/1 -> Chart/1(ValveState)
  Valve Current/1 -> Chart/2(ValveCurrent)

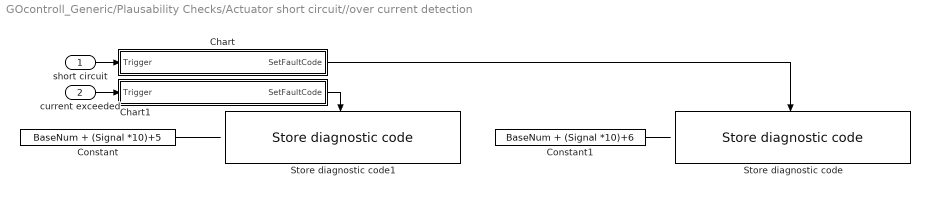
== system GOcontroll_Generic/Plausability Checks/Actuator short circuit//over current detection ==
  short circuit : Inport
  current exceeded : Inport  Port=2
  Chart : Stateflow chart  TreatAsAtomicUnit=on
  Chart1 : Stateflow chart  TreatAsAtomicUnit=on
  Constant : Constant  Value=BaseNum + (Signal *10)+5  OutDataTypeStr=uint32
  Constant1 : Constant  Value=BaseNum + (Signal *10)+6  OutDataTypeStr=uint32
  Store diagnostic code : GOcontroll_Moduline_Target/Memory store/Diagnostic to memory/Store diagnostic code  Tag=HANcoder_GOcontroll_Moduline_IV  spn=1234  fmi=(0) Data valid but above normal operational range, most severe level (3)  TriggerType=rising
      settings: SourceProductName=GOcontroll Moduline
  Store diagnostic code1 : GOcontroll_Moduline_Target/Memory store/Diagnostic to memory/Store diagnostic code  Tag=HANcoder_GOcontroll_Moduline_IV  spn=1234  fmi=(0) Data valid but above normal operational range, most severe level (3)  TriggerType=rising
      settings: SourceProductName=GOcontroll Moduline
  wires:
  Chart1/1(SetFaultCode) -> Store diagnostic code1/Trigger
  Chart/1(SetFaultCode) -> Store diagnostic code/Trigger
  Constant1/1 -> ?
  Constant/1 -> ?
  current exceeded/1 -> Chart1/1(Trigger)
  short circuit/1 -> Chart/1(Trigger)

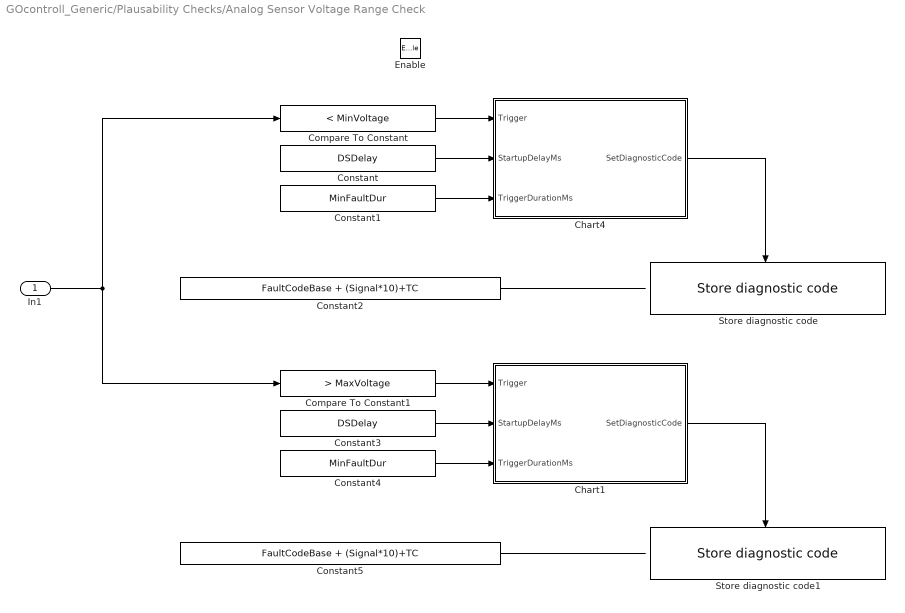
== system GOcontroll_Generic/Plausability Checks/Analog Sensor Voltage Range Check ==
  In1 : Inport
  Enable : EnablePort
  Chart1 : Stateflow chart  TreatAsAtomicUnit=on
  Chart4 : Stateflow chart  TreatAsAtomicUnit=on
  Compare To Constant : simulink/Logic and Bit Operations/Compare To Constant  relop=<  const=MinVoltage  OutDataTypeStr=boolean
  Compare To Constant1 : simulink/Logic and Bit Operations/Compare To Constant  relop=>  const=MaxVoltage  OutDataTypeStr=boolean
  Constant : Constant  Value=DSDelay  OutDataTypeStr=single
  Constant1 : Constant  Value=MinFaultDur  OutDataTypeStr=single
  Constant2 : Constant  Value=FaultCodeBase + (Signal*10)+TC  OutDataTypeStr=uint32
  Constant3 : Constant  Value=DSDelay  OutDataTypeStr=single
  Constant4 : Constant  Value=MinFaultDur  OutDataTypeStr=single
  Constant5 : Constant  Value=FaultCodeBase + (Signal*10)+TC  OutDataTypeStr=uint32
  Store diagnostic code : GOcontroll_Moduline_Target/Memory store/Diagnostic to memory/Store diagnostic code  Tag=HANcoder_GOcontroll_Moduline_IV  spn=1234  fmi=(0) Data valid but above normal operational range, most severe level (3)  TriggerType=rising
      settings: SourceProductName=GOcontroll Moduline
  Store diagnostic code1 : GOcontroll_Moduline_Target/Memory store/Diagnostic to memory/Store diagnostic code  Tag=HANcoder_GOcontroll_Moduline_IV  spn=1234  fmi=(0) Data valid but above normal operational range, most severe level (3)  TriggerType=rising
      settings: SourceProductName=GOcontroll Moduline
  wires:
  In1/1 -> Compare To Constant1/1, Compare To Constant/1
  Constant4/1 -> Chart1/3(TriggerDurationMs)
  Chart1/1(SetDiagnosticCode) -> Store diagnostic code1/Trigger
  Constant3/1 -> Chart1/2(StartupDelayMs)
  Compare To Constant1/1 -> Chart1/1(Trigger)
  Constant5/1 -> ?
  Constant2/1 -> ?
  Compare To Constant/1 -> Chart4/1(Trigger)
  Constant/1 -> Chart4/2(StartupDelayMs)
  Chart4/1(SetDiagnosticCode) -> Store diagnostic code/Trigger
  Constant1/1 -> Chart4/3(TriggerDurationMs)

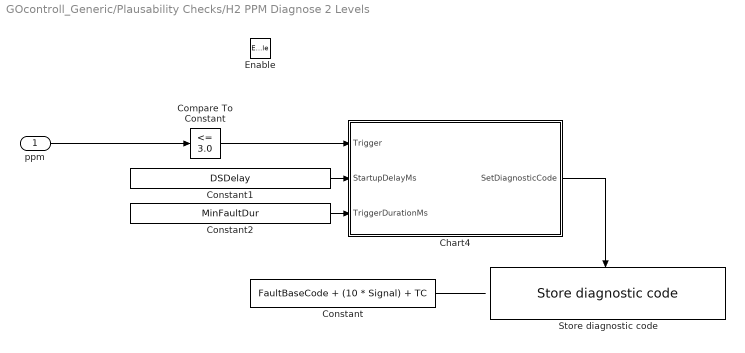
== system GOcontroll_Generic/Plausability Checks/H2 PPM Diagnose 2 Levels ==
  ppm : Inport
  Enable : EnablePort
  Chart4 : Stateflow chart  TreatAsAtomicUnit=on
  Compare To Constant : simulink/Logic and Bit Operations/Compare To Constant  relop=<=  const=3.0  OutDataTypeStr=boolean
  Constant : Constant  Value=FaultBaseCode + (10 * Signal) + TC  OutDataTypeStr=uint32
  Constant1 : Constant  Value=DSDelay  OutDataTypeStr=single
  Constant2 : Constant  Value=MinFaultDur  OutDataTypeStr=single
  Store diagnostic code : GOcontroll_Moduline_Target/Memory store/Diagnostic to memory/Store diagnostic code  Tag=HANcoder_GOcontroll_Moduline_IV  spn=1234  fmi=(0) Data valid but above normal operational range, most severe level (3)  TriggerType=rising
      settings: SourceProductName=GOcontroll Moduline
  wires:
  Constant2/1 -> Chart4/3(TriggerDurationMs)
  Constant1/1 -> Chart4/2(StartupDelayMs)
  Constant/1 -> ?
  Chart4/1(SetDiagnosticCode) -> Store diagnostic code/Trigger
  Compare To Constant/1 -> Chart4/1(Trigger)
  ppm/1 -> Compare To Constant/1

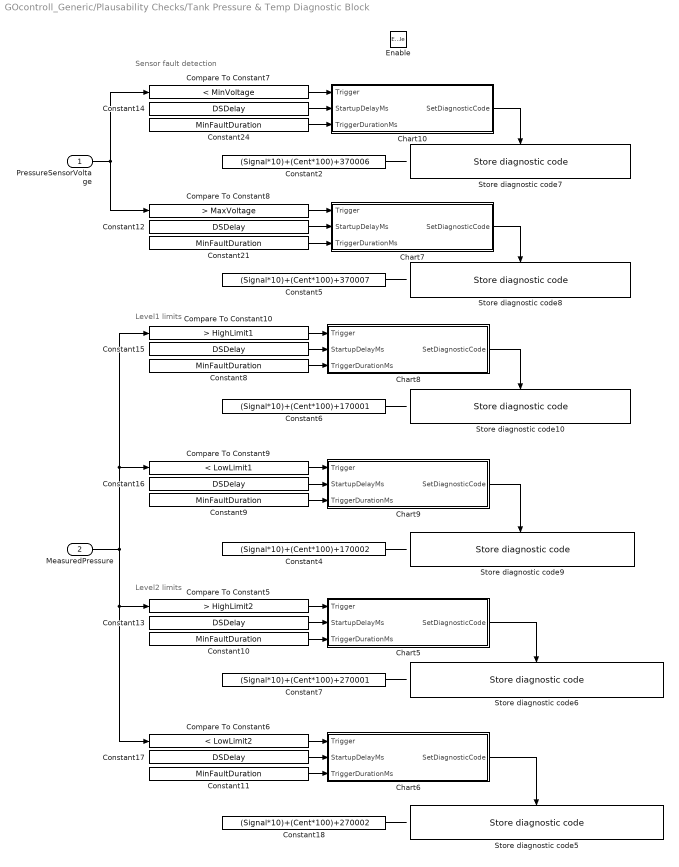
== system GOcontroll_Generic/Plausability Checks/Tank Pressure & Temp Diagnostic Block ==
  note: Level1 limits
  note: Sensor fault detection
  note: Level2 limits
  PressureSensorVoltage : Inport
  MeasuredPressure : Inport  Port=2
  Enable : EnablePort
  Chart10 : Stateflow chart  TreatAsAtomicUnit=on
  Chart5 : Stateflow chart  TreatAsAtomicUnit=on
  Chart6 : Stateflow chart  TreatAsAtomicUnit=on
  Chart7 : Stateflow chart  TreatAsAtomicUnit=on
  Chart8 : Stateflow chart  TreatAsAtomicUnit=on
  Chart9 : Stateflow chart  TreatAsAtomicUnit=on
  Compare To Constant10 : simulink/Logic and Bit Operations/Compare To Constant  relop=>  const=HighLimit1  OutDataTypeStr=boolean
  Compare To Constant5 : simulink/Logic and Bit Operations/Compare To Constant  relop=>  const=HighLimit2  OutDataTypeStr=boolean
  Compare To Constant6 : simulink/Logic and Bit Operations/Compare To Constant  relop=<  const=LowLimit2  OutDataTypeStr=boolean
  Compare To Constant7 : simulink/Logic and Bit Operations/Compare To Constant  relop=<  const=MinVoltage  OutDataTypeStr=boolean
  Compare To Constant8 : simulink/Logic and Bit Operations/Compare To Constant  relop=>  const=MaxVoltage  OutDataTypeStr=boolean
  Compare To Constant9 : simulink/Logic and Bit Operations/Compare To Constant  relop=<  const=LowLimit1  OutDataTypeStr=boolean
  Constant{8..11,21,24} (6 alike) : Constant  Value=MinFaultDuration  OutDataTypeStr=single
  Constant{12..17} (6 alike) : Constant  Value=DSDelay  OutDataTypeStr=single
  Constant18 : Constant  Value=(Signal*10)+(Cent*100)+270002  OutDataTypeStr=uint32
  Constant2 : Constant  Value=(Signal*10)+(Cent*100)+370006  OutDataTypeStr=uint32
  Constant4 : Constant  Value=(Signal*10)+(Cent*100)+170002  OutDataTypeStr=uint32
  Constant5 : Constant  Value=(Signal*10)+(Cent*100)+370007  OutDataTypeStr=uint32
  Constant6 : Constant  Value=(Signal*10)+(Cent*100)+170001  OutDataTypeStr=uint32
  Constant7 : Constant  Value=(Signal*10)+(Cent*100)+270001  OutDataTypeStr=uint32
  Store diagnostic code{5..10} (6 alike) : GOcontroll_Moduline_Target/Memory store/Diagnostic to memory/Store diagnostic code  Tag=HANcoder_GOcontroll_Moduline_IV  spn=1234  fmi=(0) Data valid but above normal operational range, most severe level (3)  TriggerType=rising
      settings: SourceProductName=GOcontroll Moduline
  wires:
  Chart5/1(SetDiagnosticCode) -> Store diagnostic code6/Trigger
  Constant15/1 -> Chart8/2(StartupDelayMs)
  Constant7/1 -> ?
  PressureSensorVoltage/1 -> Compare To Constant8/1, Compare To Constant7/1
  Constant9/1 -> Chart9/3(TriggerDurationMs)
  Constant6/1 -> ?
  Constant14/1 -> Chart10/2(StartupDelayMs)
  Constant2/1 -> ?
  Constant16/1 -> Chart9/2(StartupDelayMs)
  Constant18/1 -> ?
  Constant21/1 -> Chart7/3(TriggerDurationMs)
  Compare To Constant8/1 -> Chart7/1(Trigger)
  MeasuredPressure/1 -> Compare To Constant5/1, Compare To Constant6/1, Compare To Constant9/1, Compare To Constant10/1
  Compare To Constant6/1 -> Chart6/1(Trigger)
  Compare To Constant10/1 -> Chart8/1(Trigger)
  Constant11/1 -> Chart6/3(TriggerDurationMs)
  Compare To Constant5/1 -> Chart5/1(Trigger)
  Chart9/1(SetDiagnosticCode) -> Store diagnostic code9/Trigger
  Chart6/1(SetDiagnosticCode) -> Store diagnostic code5/Trigger
  Constant13/1 -> Chart5/2(StartupDelayMs)
  Constant4/1 -> ?
  Constant10/1 -> Chart5/3(TriggerDurationMs)
  Constant24/1 -> Chart10/3(TriggerDurationMs)
  Constant12/1 -> Chart7/2(StartupDelayMs)
  Constant17/1 -> Chart6/2(StartupDelayMs)
  Constant5/1 -> ?
  Chart10/1(SetDiagnosticCode) -> Store diagnostic code7/Trigger
  Compare To Constant7/1 -> Chart10/1(Trigger)
  Chart7/1(SetDiagnosticCode) -> Store diagnostic code8/Trigger
  Chart8/1(SetDiagnosticCode) -> Store diagnostic code10/Trigger
  Compare To Constant9/1 -> Chart9/1(Trigger)
  Constant8/1 -> Chart8/3(TriggerDurationMs)

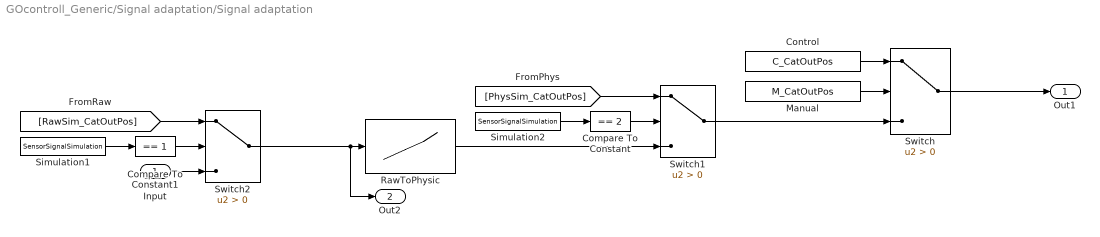
== system GOcontroll_Generic/Signal adaptation/Signal adaptation ==
  Input : Inport
  Compare To Constant : simulink/Logic and Bit Operations/Compare To Constant  relop===  const=2  OutDataTypeStr=boolean
  Compare To Constant1 : simulink/Logic and Bit Operations/Compare To Constant  relop===  const=1  OutDataTypeStr=boolean
  Control : Constant  Value=C_CatOutPos
  Manual : Constant  Value=M_CatOutPos
  RawToPhysic : Lookup_n-D  NumberOfTableDimensions=1  DataSpecification=Lookup table object  LookupTableObject=CatOutPos_Table  BreakpointsForDimension1=[-5:5]  Table=tanh([-5:5])  ExtrapMethod=Clip  InternalRulePriority=Speed  OutDataTypeStr=Inherit: Inherit from 'Table data'  RndMeth=Simplest
  Simulation1 : Constant  Value=SensorSignalSimulation
  Simulation2 : Constant  Value=SensorSignalSimulation
  Switch : Switch  Criteria=u2 > Threshold  OutDataTypeStr=single  SaturateOnIntegerOverflow=off  InputSameDT=off
  Switch1 : Switch  Criteria=u2 > Threshold  SaturateOnIntegerOverflow=off  InputSameDT=off
  Switch2 : Switch  Criteria=u2 > Threshold  SaturateOnIntegerOverflow=off  InputSameDT=off
  Out1 : Outport
  Out2 : Outport  Port=2
  wires:
  Input/1 -> Switch2/3
  [RawSim_CatOutPos] -> Switch2/1
  [PhysSim_CatOutPos] -> Switch1/1
  Simulation1/1 -> Compare To Constant1/1
  Compare To Constant1/1 -> Switch2/2
  Switch1/1 -> Switch/3
  Simulation2/1 -> Compare To Constant/1
  Compare To Constant/1 -> Switch1/2
  RawToPhysic/1 -> Switch1/3
  Switch2/1 -> RawToPhysic/1, Out2/1
  Switch/1 -> Out1/1
  Control/1 -> Switch/1
  Manual/1 -> Switch/2

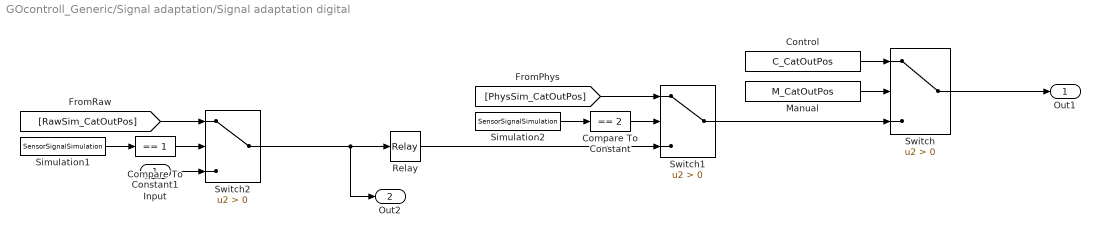
== system GOcontroll_Generic/Signal adaptation/Signal adaptation digital ==
  Input : Inport
  Compare To Constant : simulink/Logic and Bit Operations/Compare To Constant  relop===  const=2  OutDataTypeStr=boolean
  Compare To Constant1 : simulink/Logic and Bit Operations/Compare To Constant  relop===  const=1  OutDataTypeStr=boolean
  Control : Constant  Value=C_CatOutPos  OutDataTypeStr=uint8
  Manual : Constant  Value=M_CatOutPos
  Relay : Relay  OnSwitchValue=OnSwitchValue  OffSwitchValue=OffSwitchValue  OutDataTypeStr=uint8
  Simulation1 : Constant  Value=SensorSignalSimulation
  Simulation2 : Constant  Value=SensorSignalSimulation
  Switch : Switch  Criteria=u2 > Threshold  OutDataTypeStr=single  SaturateOnIntegerOverflow=off  InputSameDT=off
  Switch1 : Switch  Criteria=u2 > Threshold  SaturateOnIntegerOverflow=off  InputSameDT=off
  Switch2 : Switch  Criteria=u2 > Threshold  SaturateOnIntegerOverflow=off  InputSameDT=off
  Out1 : Outport
  Out2 : Outport  Port=2
  wires:
  Manual/1 -> Switch/2
  Control/1 -> Switch/1
  Switch/1 -> Out1/1
  Switch2/1 -> Out2/1, Relay/1
  Relay/1 -> Switch1/3
  Compare To Constant/1 -> Switch1/2
  Simulation2/1 -> Compare To Constant/1
  Switch1/1 -> Switch/3
  Compare To Constant1/1 -> Switch2/2
  Simulation1/1 -> Compare To Constant1/1
  [PhysSim_CatOutPos] -> Switch1/1
  [RawSim_CatOutPos] -> Switch2/1
  Input/1 -> Switch2/3

== system GOcontroll_Generic/Diagnostic checks/Actuator diagnostic/Per ==
  In1 : Inport
  Out1 : Outport
  wires:
  In1/1 -> Out1/1

== system GOcontroll_Generic/Diagnostic checks/Actuator diagnostic/Vol ==
  In1 : Inport
  Out1 : Outport
  wires:
  In1/1 -> Out1/1

== system GOcontroll_Generic/Diagnostic checks/Signal diagnostic/Per ==
  In1 : Inport
  Out1 : Outport
  wires:
  In1/1 -> Out1/1

== system GOcontroll_Generic/Diagnostic checks/Signal diagnostic/Vol ==
  In1 : Inport
  Out1 : Outport
  wires:
  In1/1 -> Out1/1

== stateflow chart GOcontroll_Generic/Plausability Checks/Tank Pressure & Temp Diagnostic Block/Chart8 ==
  state Entry
    en:SetDiagnosticCode = 0;
  state System_Running
  state Error_Triggered
  state Error_Triggered_Confirmed
    en:SetDiagnosticCode = 1;
  state Error_Code_Stored
    en:SetDiagnosticCode = 0;
  (default) -> Entry
  Entry -> System_Running : [after(StartupDelayMs,msec)]
  Error_Triggered -> System_Running [order 2] : [Trigger == 0]
  Error_Code_Stored -> System_Running
  System_Running -> Error_Triggered : [Trigger == 1]
  Error_Triggered -> Error_Triggered_Confirmed [order 1] : [after(TriggerDurationMs,msec)]
  Error_Triggered_Confirmed -> Error_Code_Stored : [after(1,sec)]
  data: Trigger input; StartupDelayMs input single; TriggerDurationMs input single; SetDiagnosticCode output uint8

== stateflow chart GOcontroll_Generic/Plausability Checks/Tank Pressure & Temp Diagnostic Block/Chart9 ==
  state Entry
    en:SetDiagnosticCode = 0;
  state System_Running
  state Error_Triggered
  state Error_Triggered_Confirmed
    en:SetDiagnosticCode = 1;
  state Error_Code_Stored
    en:SetDiagnosticCode = 0;
  (default) -> Entry
  Entry -> System_Running : [after(StartupDelayMs,msec)]
  Error_Triggered -> System_Running [order 2] : [Trigger == 0]
  Error_Code_Stored -> System_Running
  System_Running -> Error_Triggered : [Trigger == 1]
  Error_Triggered -> Error_Triggered_Confirmed [order 1] : [after(TriggerDurationMs,msec)]
  Error_Triggered_Confirmed -> Error_Code_Stored : [after(1,sec)]
  data: Trigger input; StartupDelayMs input single; TriggerDurationMs input single; SetDiagnosticCode output uint8

== stateflow chart GOcontroll_Generic/Plausability Checks/Analog Sensor Voltage Range Check/Chart1 ==
  state Entry
    en:SetDiagnosticCode = 0;
  state System_Running
  state Error_Triggered
  state Error_Triggered_Confirmed
    en:SetDiagnosticCode = 1;
  state Error_Code_Stored
    en:SetDiagnosticCode = 0;
  (default) -> Entry
  Entry -> System_Running : [after(StartupDelayMs,msec)]
  Error_Triggered -> System_Running [order 2] : [Trigger == 0]
  Error_Code_Stored -> System_Running
  System_Running -> Error_Triggered : [Trigger == 1]
  Error_Triggered -> Error_Triggered_Confirmed [order 1] : [after(TriggerDurationMs,msec)]
  Error_Triggered_Confirmed -> Error_Code_Stored : [after(1,sec)]
  data: Trigger input; StartupDelayMs input single; TriggerDurationMs input single; SetDiagnosticCode output uint8

== stateflow chart GOcontroll_Generic/Plausability Checks/Analog Sensor Voltage Range Check/Chart4 ==
  state Entry
    en:SetDiagnosticCode = 0;
  state System_Running
  state Error_Triggered
  state Error_Triggered_Confirmed
    en:SetDiagnosticCode = 1;
  state Error_Code_Stored
    en:SetDiagnosticCode = 0;
  (default) -> Entry
  Entry -> System_Running : [after(StartupDelayMs,msec)]
  Error_Triggered -> System_Running [order 2] : [Trigger == 0]
  Error_Code_Stored -> System_Running
  System_Running -> Error_Triggered : [Trigger == 1]
  Error_Triggered -> Error_Triggered_Confirmed [order 1] : [after(TriggerDurationMs,msec)]
  Error_Triggered_Confirmed -> Error_Code_Stored : [after(1,sec)]
  data: Trigger input; StartupDelayMs input single; TriggerDurationMs input single; SetDiagnosticCode output uint8
